simulink subsystem "get_full_tau_ref_subsys"  (R2022b)
settings: Solver=VariableStepAuto  StartTime=0.0  StopTime=10.0  RelTol=1e-3
settings Model: Creator=emu  LastModifiedBy=emu

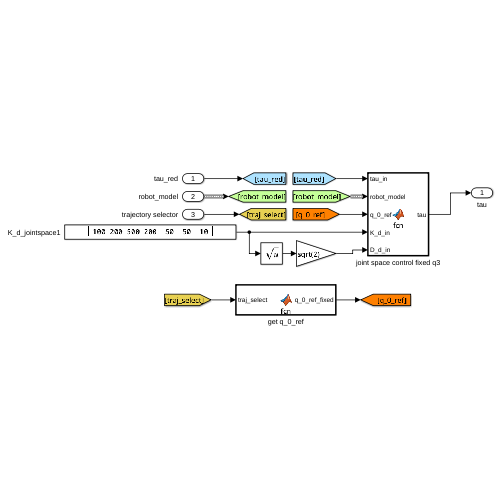
[thumbnail: Simulink's stored preview of the top-level diagram]
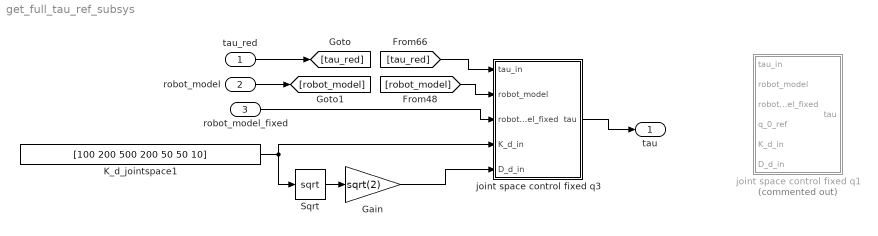
== system get_full_tau_ref_subsys ==
  tau_red : Inport
  robot_model : Inport  Port=2
  robot_model_fixed : Inport  Port=3  OutDataTypeStr=Bus: robot_model
  Gain : Gain  Gain=sqrt(2)
  K_d_jointspace1 : Constant  Value=[100 200 500 200 50 50 10]
  Sqrt : Sqrt
  joint space control fixed q1 : MATLAB Function  Commented=on  TreatAsAtomicUnit=on
  joint space control fixed q3 : MATLAB Function  TreatAsAtomicUnit=on
  tau : Outport
  wires:
  robot_model/1 -> [robot_model]
  Sqrt/1 -> Gain/1
  [robot_model] -> joint space control fixed q3/2(robot_model)
  tau_red/1 -> [tau_red]
  [tau_red] -> joint space control fixed q3/1(tau_in)
  K_d_jointspace1/1 -> Sqrt/1, joint space control fixed q3/4(K_d_in)
  Gain/1 -> joint space control fixed q3/5(D_d_in)
  joint space control fixed q3/1(tau) -> tau/1
  robot_model_fixed/1 -> joint space control fixed q3/3(robot_model_fixed)

== matlab function get_full_tau_ref_subsys/joint space control fixed q3 ==
  data: tau_in input; tau output; robot_model input Bus: robot_model; robot_model_fixed input Bus: robot_model; K_d_in input; D_d_in input; param_robot parameter
function tau = fcn(tau_in, robot_model, robot_model_fixed, K_d_in, D_d_in, param_robot)

n_indices_fixed = param_robot.n_indices_fixed;

%g = robot_model.g;
q = robot_model.q;
q_p = robot_model.q_p;

q_fix = q(n_indices_fixed); % = q3
q_p_fix = q_p(n_indices_fixed); % = q3_p
q_0_ref_fix = 0; % = q3_ref

M = robot_model_fixed.M; % mit q3 = q3_ref
C = robot_model_fixed.C; % mit q3 = q3_ref

D_d = diag(D_d_in(n_indices_fixed));
K_d = diag(K_d_in(n_indices_fixed));

A = [0 0 1 0 0 0 0];
J_psi = [eye(2) zeros(2,4); zeros(1,6); zeros(4,2) eye(4)];

M_inv = M \ eye(7);

phi = q_fix - q_0_ref_fix;
phi_p = q_p_fix;

F_psi =  tau_in;
F_phi = - A*M_inv*C*robot_model_fixed.q_p - D_d*phi_p - K_d*phi; % only here is q3

tau = [J_psi'; A*M_inv]\[F_psi;F_phi];

%tau_fix_q = M_fixed * (-K_d * (q_fix - q_0_ref_fix) -D_d*q_p_fix);
%tau_in(n_indices_fixed) = tau_in(n_indices_fixed) + tau_fix_q;
%tau = tau_in;

== matlab function get_full_tau_ref_subsys/joint space control fixed q1 ==
  data: tau_in input; tau output; robot_model input Bus: robot_model; robot_model_fixed input Bus: robot_model; q_0_ref input; K_d_in input; D_d_in input; param_robot parameter
function tau = fcn(tau_in, robot_model, robot_model_fixed, q_0_ref, K_d_in, D_d_in, param_robot)

%g = robot_model.g;
q = robot_model.q;
q_p = robot_model.q_p;
M = robot_model.M;

n_indices_fixed = param_robot.n_indices_fixed;

M_fixed = M(n_indices_fixed, n_indices_fixed);
q_0_ref_fix = q_0_ref(n_indices_fixed);

q_fix = q(n_indices_fixed);
q_p_fix = q_p(n_indices_fixed);
%g_fix = g(n_indices_fixed); is ignored

D_d = diag(D_d_in(n_indices_fixed));
K_d = diag(K_d_in(n_indices_fixed));

tau_fix_q = M_fixed * (-K_d * (q_fix - q_0_ref_fix) -D_d*q_p_fix);

tau_in(n_indices_fixed) = tau_in(n_indices_fixed) + tau_fix_q;
tau = tau_in;
